simulink model "LQR_KF_stationary"  (R2020b)
settings: Solver=ode4  StartTime=0.0  StopTime=SIM_TIME  FixedStep=STEP_SIZE  RelTol=1e-3
undefined symbols (not defined in the file): A_0, c1, c2, C_kf, f1, f2, f3, f4, f5, f6, F_kf, g, G_kf, Ki, Kx, L_kf, m, t_step, Ts, uss, V2d, xss, yss
settings Model: Creator=Roberto  LastModifiedBy=maxfi
settings DataIOCC: ReturnWorkspaceOutputs=off
settings DebuggingCC: ArithmeticOperatorsInVariantConditions=warning
settings SFSimCC: SimUseLocalCustomCode=off  CustomCodeUndefinedFunction=UseInterfaceOnly
settings RTWCC: RTWUseLocalCustomCode=off
settings CodeAppCC: StateflowObjectComments=on

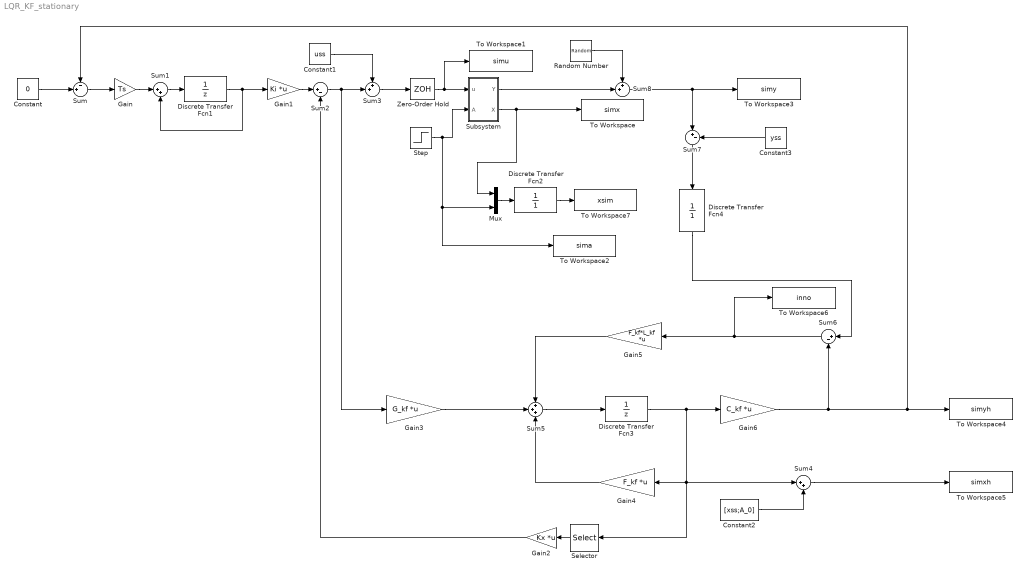
== system LQR_KF_stationary ==
  Constant : Constant  Value=0
  Constant1 : Constant  Value=uss
  Constant2 : Constant  Value=[xss;A_0]
  Constant3 : Constant  Value=yss
  Discrete Transfer Fcn1 : DiscreteTransferFcn  Denominator=[1 0]  SampleTime=Ts
  Discrete Transfer Fcn2 : DiscreteTransferFcn  Denominator=[1]  SampleTime=Ts
  Discrete Transfer Fcn3 : DiscreteTransferFcn  Denominator=[1 0]  SampleTime=Ts
  Discrete Transfer Fcn4 : DiscreteTransferFcn  Denominator=[1]  SampleTime=Ts
  Gain : Gain  Gain=Ts
  Gain1 : Gain  Gain=Ki  Multiplication=Matrix(K*u)
  Gain2 : Gain  Gain=Kx  Multiplication=Matrix(K*u)
  Gain3 : Gain  Gain=G_kf  Multiplication=Matrix(K*u)
  Gain4 : Gain  Gain=F_kf  Multiplication=Matrix(K*u)
  Gain5 : Gain  Gain=F_kf*L_kf  Multiplication=Matrix(K*u)
  Gain6 : Gain  Gain=C_kf  Multiplication=Matrix(K*u)
  Mux : Mux  Inputs=2
  Random Number : RandomNumber  Variance=V2d  SampleTime=Ts
  Selector : Selector  InputPortWidth=3  IndexOptions=Index vector (dialog)  Indices=[1 2]  OutputSizes=1
  Step : Step  Time=t_step  Before=A_0  After=A_0  SampleTime=0
  Subsystem : Subsystem
  Sum : Sum  Inputs=-+|
  Sum1 : Sum  Inputs=|++
  Sum2 : Sum  Inputs=|+-
  Sum3 : Sum  Inputs=++|
  Sum4 : Sum  Inputs=|++
  Sum5 : Sum  Inputs=+++
  Sum6 : Sum  Inputs=|+-
  Sum7 : Sum  Inputs=|+-
  Sum8 : Sum  Inputs=++|
  To Workspace : ToWorkspace  VariableName=simx  SaveFormat=Structure With Time  SampleTime=-1
  To Workspace1 : ToWorkspace  VariableName=simu  SaveFormat=Structure With Time  SampleTime=-1
  To Workspace2 : ToWorkspace  VariableName=sima  SaveFormat=Structure With Time  SampleTime=-1
  To Workspace3 : ToWorkspace  VariableName=simy  SaveFormat=Structure With Time  SampleTime=-1
  To Workspace4 : ToWorkspace  VariableName=simyh  SaveFormat=Structure With Time  SampleTime=-1
  To Workspace5 : ToWorkspace  VariableName=simxh  SaveFormat=Structure With Time  SampleTime=-1
  To Workspace6 : ToWorkspace  VariableName=inno  SaveFormat=Structure With Time  SampleTime=-1
  To Workspace7 : ToWorkspace  VariableName=xsim  SaveFormat=Structure With Time  SampleTime=-1
  Zero-Order Hold : ZeroOrderHold  SampleTime=Ts
  wires:
  Step/1 -> To Workspace2/1, Mux/2, Subsystem/2(A)
  Sum8/1 -> To Workspace3/1, Sum7/1
  Constant/1 -> Sum/2
  Gain6/1 -> To Workspace4/1, Sum/1, Sum6/2
  Sum/1 -> Gain/1
  Gain/1 -> Sum1/1
  Sum1/1 -> Discrete Transfer Fcn1/1
  Discrete Transfer Fcn1/1 -> Gain1/1, Sum1/2
  Gain1/1 -> Sum2/1
  Constant1/1 -> Sum3/1
  Sum3/1 -> Zero-Order Hold/1
  Zero-Order Hold/1 -> To Workspace1/1, Subsystem/1(u)
  Subsystem/2(X) -> Mux/1, To Workspace/1
  Discrete Transfer Fcn3/1 -> Selector/1, Sum4/1, Gain4/1, Gain6/1
  Gain2/1 -> Sum2/2
  Sum2/1 -> Gain3/1, Sum3/2
  Sum5/1 -> Discrete Transfer Fcn3/1
  Gain3/1 -> Sum5/2
  Gain4/1 -> Sum5/3
  Gain5/1 -> Sum5/1
  Sum6/1 -> To Workspace6/1, Gain5/1
  Discrete Transfer Fcn4/1 -> Sum6/1
  Constant3/1 -> Sum7/2
  Sum7/1 -> Discrete Transfer Fcn4/1
  Sum4/1 -> To Workspace5/1
  Constant2/1 -> Sum4/2
  Selector/1 -> Gain2/1
  Subsystem/1(Y) -> Sum8/2
  Random Number/1 -> Sum8/1
  Mux/1 -> Discrete Transfer Fcn2/1
  Discrete Transfer Fcn2/1 -> To Workspace7/1

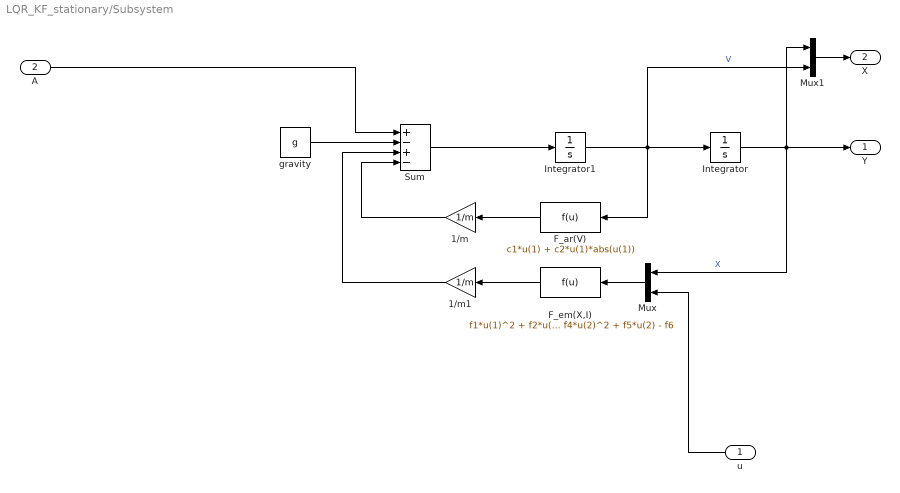
== system LQR_KF_stationary/Subsystem ==
  u : Inport
  A : Inport  Port=2
  1/m : Gain  Gain=1/m
  1/m1 : Gain  Gain=1/m
  F_ar(V) : Fcn  Expr=c1*u(1) + c2*u(1)*abs(u(1))
  F_em(X,I) : Fcn  Expr=f1*u(1)^2 + f2*u(1)*u(2) - f3*u(1) + f4*u(2)^2 + f5*u(2) - f6
  Integrator : Integrator  Priority=1  InitialCondition=xss(1)
  Integrator1 : Integrator  Priority=2  InitialCondition=xss(2)
  Mux : Mux  Inputs=2
  Mux1 : Mux  Inputs=2
  Sum : Sum  Inputs=+-+-
  gravity : Constant  Value=g
  Y : Outport
  X : Outport  Port=2
  wires:
  Integrator/1 -> Mux1/1, Y/1, Mux/1  "X"
  F_em(X,I)/1 -> 1/m1/1
  Mux/1 -> F_em(X,I)/1
  1/m1/1 -> Sum/3
  Integrator1/1 -> Mux1/2, Integrator/1, F_ar(V)/1  "V"
  gravity/1 -> Sum/2
  Sum/1 -> Integrator1/1
  1/m/1 -> Sum/4
  F_ar(V)/1 -> 1/m/1
  A/1 -> Sum/1
  u/1 -> Mux/2
  Mux1/1 -> X/1
